simulink model "water_hopper_biped_FCPG_split"  (Simulink 8.0)
settings: Solver=ode23t  StartTime=0.0  StopTime=3  MaxStep=1e-3  RelTol=1e-3
values from neighbouring files (symbols this model uses):
  alpha = 30    [SimParam_FCPG.m]
  C_d = 0.703    [SimParam_FCPG.m]
  density = 1000    [SimParam_FCPG.m]
  freq = 60    [SimParam_FCPG.m]
  g = 9.81    [SimParam_FCPG.m]
  leg_length = 0.06    [SimParam_FCPG.m]
  mass = 0.05    [SimParam_FCPG.m]
  S1 = pi*r1^2    (= 0.00125663706144)    [SimParam_FCPG.m]
  S2 = pi*r2^2    (= 7.85398163397e-05)    [SimParam_FCPG.m]
  tau = 0.001    [SimParam_FCPG.m]
undefined symbols (not defined in the file): amp, RL_lag, y_0
libraries: mblibv1 x16, simulink x1
settings Model: Creator=Metti  LastModifiedBy=Metti
settings SolverCC: ZeroCrossControl=DisableAll
settings DataIOCC: SignalLoggingSaveFormat=ModelDataLogs
settings DebuggingCC: FcnCallInpInsideContextMsg=EnableAllAsWarning
settings ConfigurationSet: Description=SimMechanics 2G

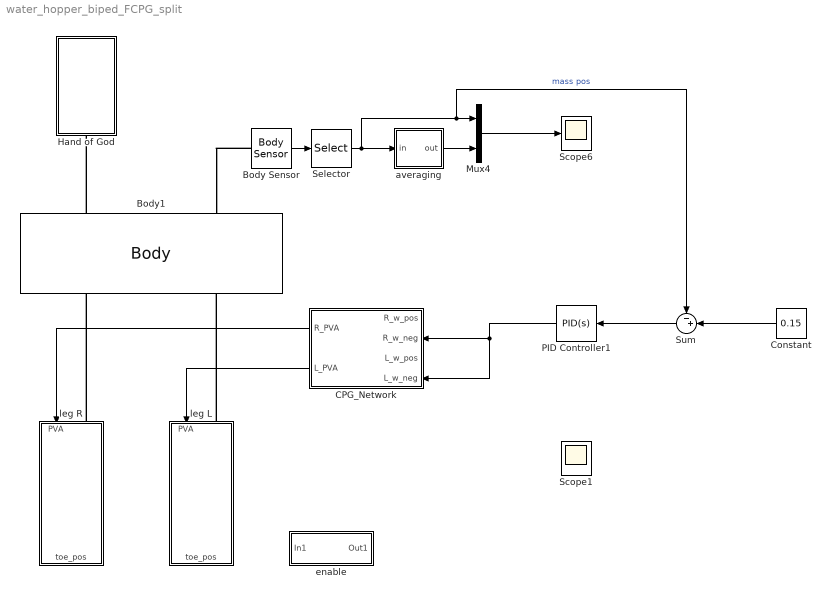
== system water_hopper_biped_FCPG_split ==
  Body Sensor : mblibv1/Sensors &  Actuators/Body Sensor  UpdateFromCAD=off  PhysicalDomain=Mechanical  PortType=blob  Muxed=on  Pose=off  Angle=on  AngleUnits=deg  ArcVelocity=off  ArcVelocityUnits=deg/s  ArcAcceleration=off  ArcAccelerationUnits=deg/s^2  CoordPosition=on  CoordPositionUnits=m  Velocity=off  VelocityUnits=m/s  Acceleration=off  AccelerationUnits=m/s^2  Quaternion=on  QuaternionDT=off  QuaternionDDT=off  QuaternionUnits=off  OutputVector=[1]  ActiveIO=on  Width=3  DialogClass=MechanicalSensorBlock  ReferenceFrame=Absolute (World)
  Body1 : mblibv1/Bodies/Body  LConnTagsString=CS1|CS2  RConnTagsString=CS3|CS4  UpdateFromCAD=off  DialogClass=MechanicalBodyBlock  Mass=mass  MassUnits=kg  InertiaUnits=kg*m^2  Inertia=eye(3)  Shape=Cylinder  ShapeDims=[1 1]  ShapeUnits=m  ShapeUse=false  Density=1  DensityUnits=kg/m^3  DensityUse=false  GraphicsMode=MACHINE_DEFAULT  BodyColorSelMode=MACHINE_DEFAULT  BodyColor=[1 0 0]  AttachedToCS=CG  CG=Left$CG$[0 0 0]$WORLD$WORLD$m$[0 0 0]$Euler X-Y-Z$deg$WORLD$false$none  WorkingFrames=Left$CS1$[0 0 0]$CG$CG$m$[0 0 0]$Euler X-Y-Z$deg$WORLD$true$none#Left$CS2$[0 0 0]$CG$CG$m$[0 0 0]$Euler X-Y-Z$deg$WORLD$true$none#Right$CS3$[0 0 0]$CG$CG$m$[0 0 0]$Euler X-Y-Z$deg$WORLD$true$none#Right$CS4$[0 0 0]$CG$CG$m$[0 0 0]$Euler X-Y-Z$deg$WORLD$true$none  CGPos=[0 0 0]  CGRot=[0 0 0]  CS0Pos=[]  CS0Rot=[]  CS1Pos=[0 0 0]  CS1Rot=[0 0 0]  CS2Pos=[0 0 0]  CS2Rot=[0 0 0]  CS3Pos=[0 0 0]  CS3Rot=[0 0 0]  CS4Pos=[0 0 0]  CS4Rot=[0 0 0]  CS5Pos=[]  CS5Rot=[]  CS6Pos=[]  CS6Rot=[]  CS7Pos=[]  CS7Rot=[]  CS8Pos=[]  CS8Rot=[]  CS9Pos=[]  CS9Rot=[]  CS10Pos=[]  CS10Rot=[]  CS11Pos=[]  CS11Rot=[]  CS12Pos=[]  CS12Rot=[]  CS13Pos=[]  CS13Rot=[]  CS14Pos=[]  CS14Rot=[]  CS15Pos=[]  CS15Rot=[]  CS16Pos=[]  CS16Rot=[]  CS17Pos=[]  CS17Rot=[]  CS18Pos=[]  CS18Rot=[]  CS19Pos=[]  CS19Rot=[]  CS20Pos=[]  CS20Rot=[]
  CPG_Network : Subsystem
  Constant : Constant  Value=0.15
  Hand of God : Subsystem
  Mux4 : Mux  Inputs=2
  PID Controller1 : simulink/Continuous/PID Controller  Controller=PID  TimeDomain=Continuous-time  SampleTime=1  IntegratorMethod=Forward Euler  FilterMethod=Forward Euler  Form=Parallel  P=100  I=0  D=0  N=100  InitialConditionSource=internal  InitialConditionForIntegrator=0  InitialConditionForFilter=0  ExternalReset=none  LimitOutput=off  UpperSaturationLimit=inf  LowerSaturationLimit=-inf  LinearizeAsGain=on  AntiWindupMode=none  Kb=1  TrackingMode=off  Kt=1  PParamMin=[]  PParamMax=[]  IParamMin=[]  IParamMax=[]  DParamMin=[]  DParamMax=[]  NParamMin=[]  NParamMax=[]  KbParamMin=[]  KbParamMax=[]  KtParamMin=[]  KtParamMax=[]  POutMin=[]  POutMax=[]  IOutMin=[]  IOutMax=[]  DOutMin=[]  DOutMax=[]  NOutMin=[]  NOutMax=[]  KbOutMin=[]  KbOutMax=[]  KtOutMin=[]  KtOutMax=[]  IntegratorOutMin=[]  IntegratorOutMax=[]  FilterOutMin=[]  FilterOutMax=[]  SumOutMin=[]  SumOutMax=[]  SumI1OutMin=[]  SumI1OutMax=[]  SumI2OutMin=[]  SumI2OutMax=[]  SumI3OutMin=[]  SumI3OutMax=[]  SumDOutMin=[]  SumDOutMax=[]  SaturationOutMin=[]  SaturationOutMax=[]  IntegratorContinuousStateAttributes=''  IntegratorStateMustResolveToSignalObject=off  IntegratorRTWStateStorageClass=Auto  FilterContinuousStateAttributes=''  FilterStateMustResolveToSignalObject=off  FilterRTWStateStorageClass=Auto
  Scope1 : Scope
      settings: YMin=0.066  YMax=0.079  SaveName=ball_position1
  Scope6 : Scope
      settings: YMin=0.066  YMax=0.079  SaveName=ball_position
  Selector : Selector  InputPortWidth=3  IndexOptions=Index vector (dialog)  Indices=[2]  OutputSizes=1
  Sum : Sum  Inputs=-+|
  averaging : Subsystem  mask{T_win=2*pi/freq/2, x_init=y_0}
      mask prompts: T_win "window (s)"; x_init "Initial condition"
  enable : Subsystem
  leg L : Subsystem
  leg R : Subsystem
  wires:
  Body Sensor/1 -> Selector/1
  Selector/1 -> averaging/1(in), Sum/1, Mux4/1  "mass pos"
  Mux4/1 -> Scope6/1
  CPG_Network/1(R_PVA) -> leg R/1(PVA)
  CPG_Network/2(L_PVA) -> leg L/1(PVA)
  Sum/1 -> PID Controller1/1
  averaging/1(out) -> Mux4/2
  Constant/1 -> Sum/2
  PID Controller1/1 -> CPG_Network/4(L_w_neg), CPG_Network/2(R_w_neg)
  connections:
  Body Sensor/LConn1 -- Body1/LConn2
  leg R/LConn1 -- Body1/RConn1
  Body1/LConn1 -- Hand of God/LConn1
  leg L/LConn1 -- Body1/RConn2

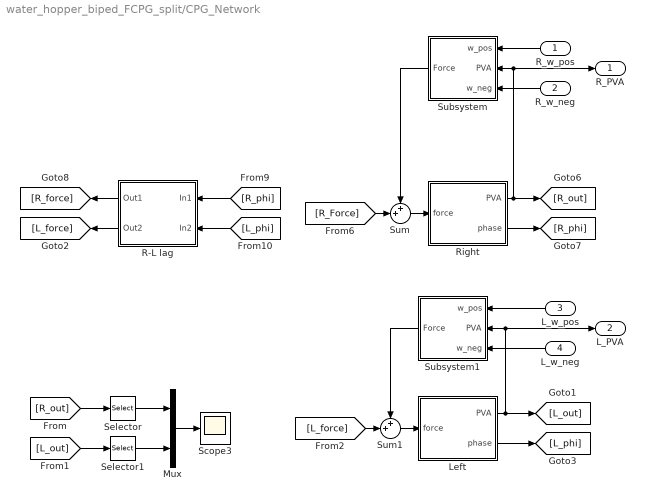
== system water_hopper_biped_FCPG_split/CPG_Network ==
  R_w_neg : Inport  Port=2
  L_w_pos : Inport  Port=3
  L_w_neg : Inport  Port=4
  Left : Subsystem  mask{Amp=amp, Offset=0, init_phi=pi}
      mask prompts: Amp "Amplitude"; init_phi "Initial Phase"
  Mux : Mux  Inputs=2
  R-L lag : Subsystem  mask{d_phase=RL_lag, coupling_weight=2}
      mask prompts: d_phase "Phase Lag"; coupling_weight "Coupling Weight"
  Right : Subsystem  mask{Amp=amp, Offset=0, init_phi=0}
      mask prompts: Amp "Amplitude"; init_phi "Initial Phase"
  Scope3 : Scope
      settings: TimeRange=10  YMin=0  YMax=2  SaveName=Output
  Selector : Selector  InputPortWidth=3  IndexOptions=Index vector (dialog)  Indices=[1]  OutputSizes=1
  Selector1 : Selector  InputPortWidth=3  IndexOptions=Index vector (dialog)  Indices=[1]  OutputSizes=1
  Sum : Sum  Inputs=++|
  Sum1 : Sum  Inputs=++|
  R_w_pos : Inport
  Subsystem : Subsystem
  Subsystem1 : Subsystem
  R_PVA : Outport
  L_PVA : Outport  Port=2
  wires:
  Mux/1 -> Scope3/1
  Left/2(phase) -> [L_phi]
  Right/2(phase) -> [R_phi]
  [L_phi] -> R-L lag/2(In2)
  [R_phi] -> R-L lag/1(In1)
  R-L lag/1(Out1) -> [R_force]
  R-L lag/2(Out2) -> [L_force]
  Right/1(PVA) -> R_PVA/1, Subsystem/2(PVA), [R_out]
  [L_force] -> Sum1/2
  Sum1/1 -> Left/1(force)
  Sum/1 -> Right/1(force)
  [R_Force] -> Sum/2
  [L_out] -> Selector1/1
  Selector1/1 -> Mux/2
  Selector/1 -> Mux/1
  [R_out] -> Selector/1
  R_w_pos/1 -> Subsystem/1(w_pos)
  R_w_neg/1 -> Subsystem/3(w_neg)
  Subsystem/1(Force) -> Sum/1
  L_w_pos/1 -> Subsystem1/1(w_pos)
  L_w_neg/1 -> Subsystem1/3(w_neg)
  Left/1(PVA) -> Subsystem1/2(PVA), L_PVA/1, [L_out]
  Subsystem1/1(Force) -> Sum1/1

== system water_hopper_biped_FCPG_split/Hand of God ==
  Ground : mblibv1/Bodies/Ground  UpdateFromCAD=off  LeftPortType=env  RightPortType=workingframe  PhysicalDomain=Mechanical  DialogClass=GroundBlock  CoordPosition=[0 0 0]  CoordPositionUnits=m  StateVectorMgrId=2  MachineId=[3 0]  ShowEnvPort=on
  Joint Initial Condition : mblibv1/Sensors &  Actuators/Joint Initial Condition  UpdateFromCAD=off  LeftPortType=blob  RightPortType=blob  PhysicalDomain=mechanical  DialogClass=InitialConditionBlock  InitialConditions=P1$true$y_0$m$deg$0$m/s$deg/s#P2$false$0$m$deg$0$m/s$deg/s#P3$false$0$m$deg$0$m/s$deg/s#R1$false$0$m$deg$0$m/s$deg/s#R2$false$0$m$deg$0$m/s$deg/s#R3$false$0$m$deg$0$m/s$deg/s#S$false$0$m$deg$0$m/s$deg/s  P1PIC=y_0  P1VIC=0  P2PIC=0  P2VIC=0  P3PIC=0  P3VIC=0  R1PIC=0  R1VIC=0  R2PIC=0  R2VIC=0  R3PIC=0  R3VIC=0  SPIC=0  SVIC=0
  Machine Environment : mblibv1/Bodies/Machine Environment  PortType=env  PhysicalDomain=Mechanical  DialogTemplateClass=MECH.MachineEnvironment  SyncWhenCopied=off  Gravity=[0 -g 0]  GravityUnits=m/s^2  GravityAsSignal=off  Dimensionality=Auto-detect  AnalysisType=Forward dynamics  LinearAssemblyTolerance=1e-3  LinearAssemblyToleranceUnits=m  AngularAssemblyTolerance=1e-3  AngularAssemblyToleranceUnits=rad  ConstraintSolverType=Stabilizing  ConstraintRelTolerance=1e-4  ConstraintAbsTolerance=1e-4  UseRobustSingularityHandling=off  RedundancyAnalysisToleranceType=Automatically select tolerance  RedundancyAnalysisTolerance=1e-14  StatePerturbationType=Fixed  PerturbationSize=1e-5  VisualizeMachine=on  BodyVisualizationType=Use model default body geometries  BodyColorSelMode=Use model default  DefaultBodyColor=[1 0 0]
  Prismatic : mblibv1/Joints/Prismatic  LConnTagsString=__newl0|SA1  RConnTagsString=__newr0  UpdateFromCAD=off  NumSAPorts=1  CutJoint=off  MarkAsCut=off  Primitives=prismatic  PrimitiveProps=P1$World$[0 1 0]$prismatic  DialogClass=JointBlock  P1Axis=[0 1 0]
  Conn1 : PMIOPort  Port=1  Side=Left
  connections:
  Conn1/RConn1 -- Prismatic/RConn1
  Machine Environment/RConn1 -- Ground/LConn1
  Ground/RConn1 -- Prismatic/LConn1
  Joint Initial Condition/RConn1 -- Prismatic/LConn2

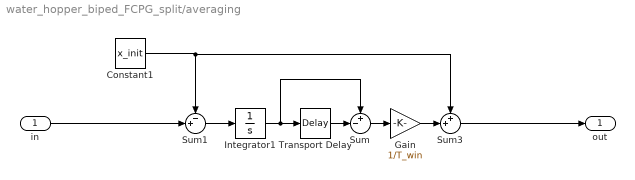
== system water_hopper_biped_FCPG_split/averaging ==
  in : Inport
  Constant1 : Constant  Value=x_init
  Gain : Gain  Gain=1/T_win
  Integrator1 : Integrator
  Sum : Sum  Inputs=+-|
  Sum1 : Sum  Inputs=-+|
  Sum3 : Sum  Inputs=++|
  Transport Delay : TransportDelay  DelayTime=T_win
  out : Outport
  wires:
  in/1 -> Sum1/2
  Gain/1 -> Sum3/2
  Constant1/1 -> Sum3/1, Sum1/1
  Sum1/1 -> Integrator1/1
  Transport Delay/1 -> Sum/2
  Integrator1/1 -> Sum/1, Transport Delay/1
  Sum3/1 -> out/1
  Sum/1 -> Gain/1

== system water_hopper_biped_FCPG_split/enable ==
  In1 : Inport
  Constant1 : Constant
  Derivative : Derivative
  Gain : Gain  Gain=.5
  Sign : Signum
  Sum1 : Sum  Inputs=|-+
  Out1 : Outport
  wires:
  Derivative/1 -> Sign/1
  Constant1/1 -> Sum1/2
  Sign/1 -> Sum1/1
  Gain/1 -> Out1/1
  In1/1 -> Derivative/1
  Sum1/1 -> Gain/1

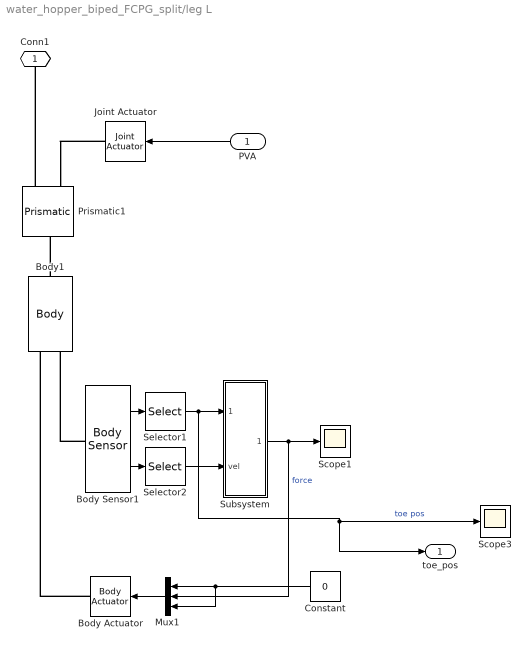
== system water_hopper_biped_FCPG_split/leg L ==
  PVA : Inport
  Body Actuator : mblibv1/Sensors &  Actuators/Body Actuator  UpdateFromCAD=off  PhysicalDomain=Mechanical  PortType=blob  ActuationStyle=Force  AngleUnits=deg  ArcVelocityUnits=deg/s  ArcAccelerationUnits=deg/s^2  CoordPositionUnits=m  VelocityUnits=m/s  AccelerationUnits=m/s^2  ForceUnits=N  TorqueUnits=N-m  ActiveIO=on  Width=3  DialogClass=MechanicalActuatorBlock  ReferenceFrame=Absolute (World)  Angle=off  CoordPosition=on  Force=on  Torque=off
  Body Sensor1 : mblibv1/Sensors &  Actuators/Body Sensor  UpdateFromCAD=off  PhysicalDomain=Mechanical  PortType=blob  Muxed=off  Pose=off  Angle=on  AngleUnits=deg  ArcVelocity=off  ArcVelocityUnits=deg/s  ArcAcceleration=off  ArcAccelerationUnits=deg/s^2  CoordPosition=on  CoordPositionUnits=m  Velocity=on  VelocityUnits=m/s  Acceleration=off  AccelerationUnits=m/s^2  Quaternion=on  QuaternionDT=off  QuaternionDDT=off  QuaternionUnits=off  OutputVector=[1]  ActiveIO=on  Width=6  DialogClass=MechanicalSensorBlock  ReferenceFrame=Absolute (World)
  Body1 : mblibv1/Bodies/Body  LConnTagsString=CS1  RConnTagsString=CS2|CS3  UpdateFromCAD=off  DialogClass=MechanicalBodyBlock  Mass=0  MassUnits=kg  InertiaUnits=kg*m^2  Inertia=zeros(3)  Shape=Cylinder  ShapeDims=[1 1]  ShapeUnits=m  ShapeUse=false  Density=1  DensityUnits=kg/m^3  DensityUse=false  GraphicsMode=MACHINE_DEFAULT  BodyColorSelMode=MACHINE_DEFAULT  BodyColor=[1 0 0]  AttachedToCS=CG  CG=Left$CG$[0 -leg_length 0]$CS1$CS1$m$[0 0 0]$Euler X-Y-Z$deg$WORLD$false$none  WorkingFrames=Left$CS1$[0 0 0]$Adjoining$Adjoining$m$[0 0 0]$Euler X-Y-Z$deg$WORLD$true$none#Right$CS2$[0 -leg_length 0]$CS1$CS1$m$[0 0 0]$Euler X-Y-Z$deg$WORLD$true$none#Right$CS3$[0 -leg_length 0]$CS1$CS1$m$[0 0 0]$Euler X-Y-Z$deg$WORLD$true$none  CGPos=[0 -leg_length 0]  CGRot=[0 0 0]  CS0Pos=[]  CS0Rot=[]  CS1Pos=[0 0 0]  CS1Rot=[0 0 0]  CS2Pos=[0 -leg_length 0]  CS2Rot=[0 0 0]  CS3Pos=[0 -leg_length 0]  CS3Rot=[0 0 0]  CS4Pos=[]  CS4Rot=[]  CS5Pos=[]  CS5Rot=[]  CS6Pos=[]  CS6Rot=[]  CS7Pos=[]  CS7Rot=[]  CS8Pos=[]  CS8Rot=[]  CS9Pos=[]  CS9Rot=[]  CS10Pos=[]  CS10Rot=[]  CS11Pos=[]  CS11Rot=[]  CS12Pos=[]  CS12Rot=[]  CS13Pos=[]  CS13Rot=[]  CS14Pos=[]  CS14Rot=[]  CS15Pos=[]  CS15Rot=[]  CS16Pos=[]  CS16Rot=[]  CS17Pos=[]  CS17Rot=[]  CS18Pos=[]  CS18Rot=[]  CS19Pos=[]  CS19Rot=[]  CS20Pos=[]  CS20Rot=[]
  Constant : Constant  Value=0
  Joint Actuator : mblibv1/Sensors &  Actuators/Joint Actuator  UpdateFromCAD=off  PhysicalDomain=Mechanical  PortType=blob  ActuationStyle=Motion  AngleUnits=deg  ArcVelocityUnits=deg/s  ArcAccelerationUnits=deg/s^2  CoordPositionUnits=m  VelocityUnits=m/s  AccelerationUnits=m/s^2  ForceUnits=N  TorqueUnits=N*m  ActiveIO=on  Width=3  DialogClass=MechanicalActuatorBlock  Primitive=P1  ReferenceFrame=Absolute (World)
  Mux1 : Mux  Inputs=3
  Prismatic1 : mblibv1/Joints/Prismatic  LConnTagsString=__newl0|SA1  RConnTagsString=__newr0  UpdateFromCAD=off  NumSAPorts=1  CutJoint=off  MarkAsCut=off  Primitives=prismatic  PrimitiveProps=P1$World$[0 1 0]$prismatic  DialogClass=JointBlock  P1Axis=[0 1 0]
  Scope1 : Scope
      settings: SaveName=force_L
  Scope3 : Scope
      settings: SaveName=toe_position_L
  Selector1 : Selector  InputPortWidth=3  IndexOptions=Index vector (dialog)  Indices=[2]  OutputSizes=1
  Selector2 : Selector  InputPortWidth=3  IndexOptions=Index vector (dialog)  Indices=[2]  OutputSizes=1
  Subsystem : Subsystem
  Conn1 : PMIOPort  Port=1  Side=Left
  toe_pos : Outport
  wires:
  PVA/1 -> Joint Actuator/1
  Constant/1 -> Mux1/3, Mux1/1
  Mux1/1 -> Body Actuator/1
  Subsystem/1(force) -> Mux1/2, Scope1/1  "force"
  Selector2/1 -> Subsystem/2(vel)
  Selector1/1 -> toe_pos/1, Scope3/1, Subsystem/1(pos)  "toe pos"
  Body Sensor1/2 -> Selector2/1
  Body Sensor1/1 -> Selector1/1
  connections:
  Joint Actuator/RConn1 -- Prismatic1/LConn2
  Prismatic1/LConn1 -- Conn1/RConn1
  Body Sensor1/LConn1 -- Body1/RConn2
  Body Actuator/RConn1 -- Body1/RConn1
  Body1/LConn1 -- Prismatic1/RConn1

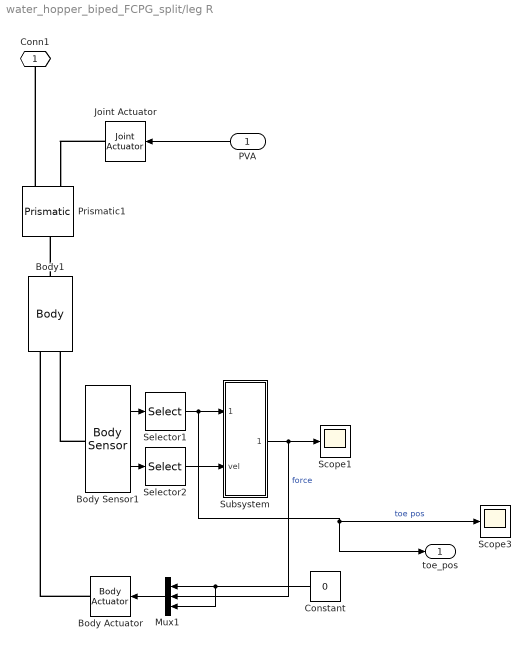
== system water_hopper_biped_FCPG_split/leg R ==
  PVA : Inport
  Body Actuator : mblibv1/Sensors &  Actuators/Body Actuator  UpdateFromCAD=off  PhysicalDomain=Mechanical  PortType=blob  ActuationStyle=Force  AngleUnits=deg  ArcVelocityUnits=deg/s  ArcAccelerationUnits=deg/s^2  CoordPositionUnits=m  VelocityUnits=m/s  AccelerationUnits=m/s^2  ForceUnits=N  TorqueUnits=N-m  ActiveIO=on  Width=3  DialogClass=MechanicalActuatorBlock  ReferenceFrame=Absolute (World)  Angle=off  CoordPosition=on  Force=on  Torque=off
  Body Sensor1 : mblibv1/Sensors &  Actuators/Body Sensor  UpdateFromCAD=off  PhysicalDomain=Mechanical  PortType=blob  Muxed=off  Pose=off  Angle=on  AngleUnits=deg  ArcVelocity=off  ArcVelocityUnits=deg/s  ArcAcceleration=off  ArcAccelerationUnits=deg/s^2  CoordPosition=on  CoordPositionUnits=m  Velocity=on  VelocityUnits=m/s  Acceleration=off  AccelerationUnits=m/s^2  Quaternion=on  QuaternionDT=off  QuaternionDDT=off  QuaternionUnits=off  OutputVector=[1]  ActiveIO=on  Width=6  DialogClass=MechanicalSensorBlock  ReferenceFrame=Absolute (World)
  Body1 : mblibv1/Bodies/Body  LConnTagsString=CS1  RConnTagsString=CS2|CS3  UpdateFromCAD=off  DialogClass=MechanicalBodyBlock  Mass=0  MassUnits=kg  InertiaUnits=kg*m^2  Inertia=zeros(3)  Shape=Cylinder  ShapeDims=[1 1]  ShapeUnits=m  ShapeUse=false  Density=1  DensityUnits=kg/m^3  DensityUse=false  GraphicsMode=MACHINE_DEFAULT  BodyColorSelMode=MACHINE_DEFAULT  BodyColor=[1 0 0]  AttachedToCS=CG  CG=Left$CG$[0 -leg_length 0]$CS1$CS1$m$[0 0 0]$Euler X-Y-Z$deg$WORLD$false$none  WorkingFrames=Left$CS1$[0 0 0]$Adjoining$Adjoining$m$[0 0 0]$Euler X-Y-Z$deg$WORLD$true$none#Right$CS2$[0 -leg_length 0]$CS1$CS1$m$[0 0 0]$Euler X-Y-Z$deg$WORLD$true$none#Right$CS3$[0 -leg_length 0]$CS1$CS1$m$[0 0 0]$Euler X-Y-Z$deg$WORLD$true$none  CGPos=[0 -leg_length 0]  CGRot=[0 0 0]  CS0Pos=[]  CS0Rot=[]  CS1Pos=[0 0 0]  CS1Rot=[0 0 0]  CS2Pos=[0 -leg_length 0]  CS2Rot=[0 0 0]  CS3Pos=[0 -leg_length 0]  CS3Rot=[0 0 0]  CS4Pos=[]  CS4Rot=[]  CS5Pos=[]  CS5Rot=[]  CS6Pos=[]  CS6Rot=[]  CS7Pos=[]  CS7Rot=[]  CS8Pos=[]  CS8Rot=[]  CS9Pos=[]  CS9Rot=[]  CS10Pos=[]  CS10Rot=[]  CS11Pos=[]  CS11Rot=[]  CS12Pos=[]  CS12Rot=[]  CS13Pos=[]  CS13Rot=[]  CS14Pos=[]  CS14Rot=[]  CS15Pos=[]  CS15Rot=[]  CS16Pos=[]  CS16Rot=[]  CS17Pos=[]  CS17Rot=[]  CS18Pos=[]  CS18Rot=[]  CS19Pos=[]  CS19Rot=[]  CS20Pos=[]  CS20Rot=[]
  Constant : Constant  Value=0
  Joint Actuator : mblibv1/Sensors &  Actuators/Joint Actuator  UpdateFromCAD=off  PhysicalDomain=Mechanical  PortType=blob  ActuationStyle=Motion  AngleUnits=deg  ArcVelocityUnits=deg/s  ArcAccelerationUnits=deg/s^2  CoordPositionUnits=m  VelocityUnits=m/s  AccelerationUnits=m/s^2  ForceUnits=N  TorqueUnits=N*m  ActiveIO=on  Width=3  DialogClass=MechanicalActuatorBlock  Primitive=P1  ReferenceFrame=Absolute (World)
  Mux1 : Mux  Inputs=3
  Prismatic1 : mblibv1/Joints/Prismatic  LConnTagsString=__newl0|SA1  RConnTagsString=__newr0  UpdateFromCAD=off  NumSAPorts=1  CutJoint=off  MarkAsCut=off  Primitives=prismatic  PrimitiveProps=P1$World$[0 1 0]$prismatic  DialogClass=JointBlock  P1Axis=[0 1 0]
  Scope1 : Scope
      settings: SaveName=force_L
  Scope3 : Scope
      settings: SaveName=toe_position_L
  Selector1 : Selector  InputPortWidth=3  IndexOptions=Index vector (dialog)  Indices=[2]  OutputSizes=1
  Selector2 : Selector  InputPortWidth=3  IndexOptions=Index vector (dialog)  Indices=[2]  OutputSizes=1
  Subsystem : Subsystem
  Conn1 : PMIOPort  Port=1  Side=Left
  toe_pos : Outport
  wires:
  Body Sensor1/1 -> Selector1/1
  Body Sensor1/2 -> Selector2/1
  Selector1/1 -> Subsystem/1(pos), Scope3/1, toe_pos/1  "toe pos"
  Selector2/1 -> Subsystem/2(vel)
  Subsystem/1(force) -> Scope1/1, Mux1/2  "force"
  Mux1/1 -> Body Actuator/1
  Constant/1 -> Mux1/1, Mux1/3
  PVA/1 -> Joint Actuator/1
  connections:
  Body1/LConn1 -- Prismatic1/RConn1
  Body Actuator/RConn1 -- Body1/RConn1
  Body Sensor1/LConn1 -- Body1/RConn2
  Prismatic1/LConn1 -- Conn1/RConn1
  Joint Actuator/RConn1 -- Prismatic1/LConn2

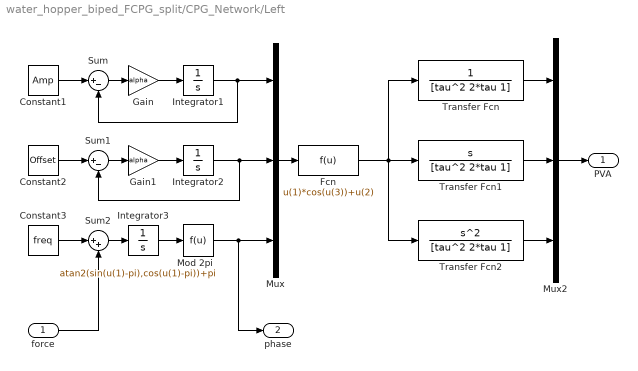
== system water_hopper_biped_FCPG_split/CPG_Network/Left ==
  force : Inport
  Constant1 : Constant  Value=Amp
  Constant2 : Constant  Value=Offset
  Constant3 : Constant  Value=freq
  Fcn : Fcn  Expr=u(1)*cos(u(3))+u(2)
  Gain : Gain  Gain=alpha
  Gain1 : Gain  Gain=alpha
  Integrator1 : Integrator
  Integrator2 : Integrator
  Integrator3 : Integrator  InitialCondition=init_phi + 0.01*rand
  Mod 2pi : Fcn  Expr=atan2(sin(u(1)-pi),cos(u(1)-pi))+pi
  Mux : Mux  Inputs=3
  Mux2 : Mux  Inputs=3
  Sum : Sum  Inputs=|+-
  Sum1 : Sum  Inputs=|+-
  Sum2 : Sum  Inputs=|++
  Transfer Fcn : TransferFcn  Denominator=[tau^2 2*tau 1]
  Transfer Fcn1 : TransferFcn  Numerator=[1 0]  Denominator=[tau^2 2*tau 1]
  Transfer Fcn2 : TransferFcn  Numerator=[1 0 0]  Denominator=[tau^2 2*tau 1]
  PVA : Outport
  phase : Outport  Port=2
  wires:
  Mux2/1 -> PVA/1
  Fcn/1 -> Transfer Fcn1/1, Transfer Fcn/1, Transfer Fcn2/1
  Transfer Fcn1/1 -> Mux2/2
  Transfer Fcn/1 -> Mux2/1
  Transfer Fcn2/1 -> Mux2/3
  force/1 -> Sum2/2
  Sum2/1 -> Integrator3/1
  Constant3/1 -> Sum2/1
  Integrator3/1 -> Mod 2pi/1
  Mod 2pi/1 -> Mux/3, phase/1
  Mux/1 -> Fcn/1
  Gain1/1 -> Integrator2/1
  Constant2/1 -> Sum1/1
  Integrator2/1 -> Mux/2, Sum1/2
  Sum1/1 -> Gain1/1
  Gain/1 -> Integrator1/1
  Constant1/1 -> Sum/1
  Integrator1/1 -> Mux/1, Sum/2
  Sum/1 -> Gain/1

== system water_hopper_biped_FCPG_split/CPG_Network/R-L lag ==
  In1 : Inport
  In2 : Inport  Port=2
  Constant : Constant  Value=d_phase
  Gain : Gain  Gain=-1
  Sum : Sum  Inputs=--+
  sin : Fcn  Expr=coupling_weight*sin(u(1))
  Out1 : Outport
  Out2 : Outport  Port=2
  wires:
  Sum/1 -> sin/1
  sin/1 -> Gain/1, Out1/1
  Constant/1 -> Sum/2
  In1/1 -> Sum/1
  In2/1 -> Sum/3
  Gain/1 -> Out2/1

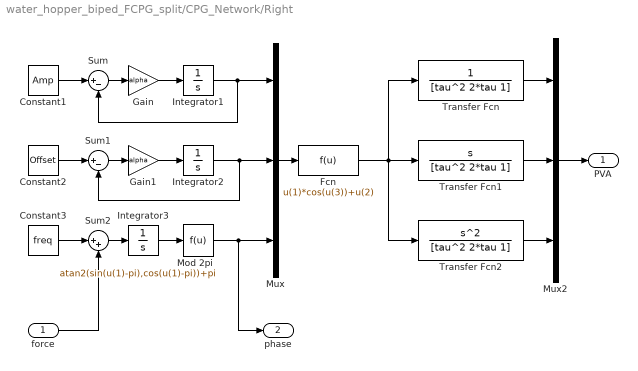
== system water_hopper_biped_FCPG_split/CPG_Network/Right ==
  force : Inport
  Constant1 : Constant  Value=Amp
  Constant2 : Constant  Value=Offset
  Constant3 : Constant  Value=freq
  Fcn : Fcn  Expr=u(1)*cos(u(3))+u(2)
  Gain : Gain  Gain=alpha
  Gain1 : Gain  Gain=alpha
  Integrator1 : Integrator
  Integrator2 : Integrator
  Integrator3 : Integrator  InitialCondition=init_phi + 0.01*rand
  Mod 2pi : Fcn  Expr=atan2(sin(u(1)-pi),cos(u(1)-pi))+pi
  Mux : Mux  Inputs=3
  Mux2 : Mux  Inputs=3
  Sum : Sum  Inputs=|+-
  Sum1 : Sum  Inputs=|+-
  Sum2 : Sum  Inputs=|++
  Transfer Fcn : TransferFcn  Denominator=[tau^2 2*tau 1]
  Transfer Fcn1 : TransferFcn  Numerator=[1 0]  Denominator=[tau^2 2*tau 1]
  Transfer Fcn2 : TransferFcn  Numerator=[1 0 0]  Denominator=[tau^2 2*tau 1]
  PVA : Outport
  phase : Outport  Port=2
  wires:
  Sum/1 -> Gain/1
  Integrator1/1 -> Sum/2, Mux/1
  Constant1/1 -> Sum/1
  Gain/1 -> Integrator1/1
  Sum1/1 -> Gain1/1
  Integrator2/1 -> Sum1/2, Mux/2
  Constant2/1 -> Sum1/1
  Gain1/1 -> Integrator2/1
  Mux/1 -> Fcn/1
  Mod 2pi/1 -> phase/1, Mux/3
  Integrator3/1 -> Mod 2pi/1
  Constant3/1 -> Sum2/1
  Sum2/1 -> Integrator3/1
  force/1 -> Sum2/2
  Transfer Fcn2/1 -> Mux2/3
  Transfer Fcn/1 -> Mux2/1
  Transfer Fcn1/1 -> Mux2/2
  Fcn/1 -> Transfer Fcn2/1, Transfer Fcn/1, Transfer Fcn1/1
  Mux2/1 -> PVA/1

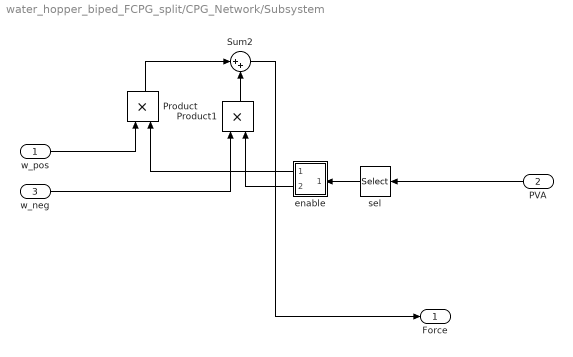
== system water_hopper_biped_FCPG_split/CPG_Network/Subsystem ==
  w_pos : Inport
  PVA : Inport  Port=2
  w_neg : Inport  Port=3
  Product : Product  RndMeth=Zero
  Product1 : Product  RndMeth=Zero
  Sum2 : Sum  Inputs=|++
  enable : Subsystem
  sel : Selector  InputPortWidth=3  IndexOptions=Index vector (dialog)  Indices=[2]  OutputSizes=1
  Force : Outport
  wires:
  Product/1 -> Sum2/1
  w_pos/1 -> Product/1
  w_neg/1 -> Product1/1
  Product1/1 -> Sum2/2
  PVA/1 -> sel/1
  enable/1(pos) -> Product/2
  enable/2(neg) -> Product1/2
  Sum2/1 -> Force/1
  sel/1 -> enable/1(in)

== system water_hopper_biped_FCPG_split/CPG_Network/Subsystem1 ==
  w_pos : Inport
  PVA : Inport  Port=2
  w_neg : Inport  Port=3
  Product : Product  RndMeth=Zero
  Product1 : Product  RndMeth=Zero
  Sum2 : Sum  Inputs=|++
  enable : Subsystem
  sel : Selector  InputPortWidth=3  IndexOptions=Index vector (dialog)  Indices=[2]  OutputSizes=1
  Force : Outport
  wires:
  Product/1 -> Sum2/1
  w_pos/1 -> Product/1
  w_neg/1 -> Product1/1
  Product1/1 -> Sum2/2
  PVA/1 -> sel/1
  enable/1(pos) -> Product/2
  enable/2(neg) -> Product1/2
  Sum2/1 -> Force/1
  sel/1 -> enable/1(in)

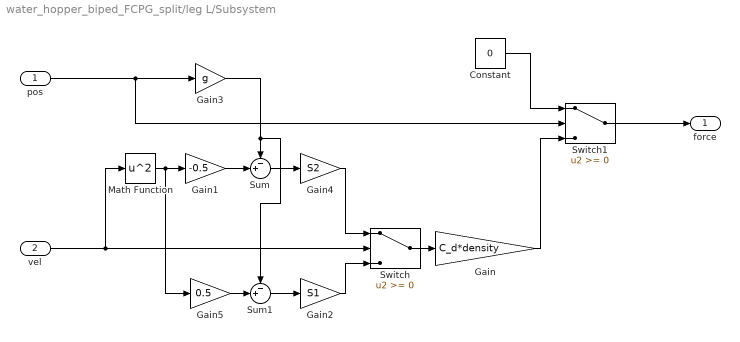
== system water_hopper_biped_FCPG_split/leg L/Subsystem ==
  pos : Inport
  vel : Inport  Port=2
  Constant : Constant  Value=0
  Gain : Gain  Gain=C_d*density
  Gain1 : Gain  Gain=-0.5
  Gain2 : Gain  Gain=S1
  Gain3 : Gain  Gain=g
  Gain4 : Gain  Gain=S2
  Gain5 : Gain  Gain=0.5
  Math Function : Math  Operator=square  SaturateOnIntegerOverflow=on
  Sum : Sum  Inputs=-+|
  Sum1 : Sum  Inputs=-+|
  Switch : Switch  ZeroCross=off
  Switch1 : Switch
  force : Outport
  wires:
  Gain5/1 -> Sum1/2
  Sum1/1 -> Gain2/1
  Constant/1 -> Switch1/1
  Gain/1 -> Switch1/3
  Switch1/1 -> force/1
  Switch/1 -> Gain/1
  Gain2/1 -> Switch/3
  Gain4/1 -> Switch/1
  Sum/1 -> Gain4/1
  Gain3/1 -> Sum1/1, Sum/1
  pos/1 -> Switch1/2, Gain3/1
  Gain1/1 -> Sum/2
  Math Function/1 -> Gain5/1, Gain1/1
  vel/1 -> Math Function/1, Switch/2

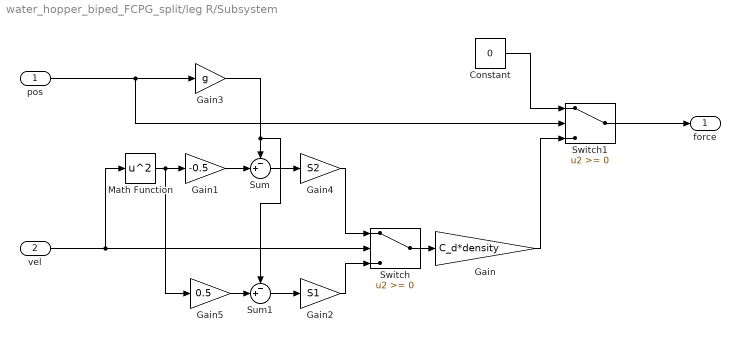
== system water_hopper_biped_FCPG_split/leg R/Subsystem ==
  pos : Inport
  vel : Inport  Port=2
  Constant : Constant  Value=0
  Gain : Gain  Gain=C_d*density
  Gain1 : Gain  Gain=-0.5
  Gain2 : Gain  Gain=S1
  Gain3 : Gain  Gain=g
  Gain4 : Gain  Gain=S2
  Gain5 : Gain  Gain=0.5
  Math Function : Math  Operator=square  SaturateOnIntegerOverflow=on
  Sum : Sum  Inputs=-+|
  Sum1 : Sum  Inputs=-+|
  Switch : Switch  ZeroCross=off
  Switch1 : Switch
  force : Outport
  wires:
  vel/1 -> Switch/2, Math Function/1
  Math Function/1 -> Gain1/1, Gain5/1
  Gain1/1 -> Sum/2
  pos/1 -> Gain3/1, Switch1/2
  Gain3/1 -> Sum/1, Sum1/1
  Sum/1 -> Gain4/1
  Gain4/1 -> Switch/1
  Gain2/1 -> Switch/3
  Switch/1 -> Gain/1
  Switch1/1 -> force/1
  Gain/1 -> Switch1/3
  Constant/1 -> Switch1/1
  Sum1/1 -> Gain2/1
  Gain5/1 -> Sum1/2

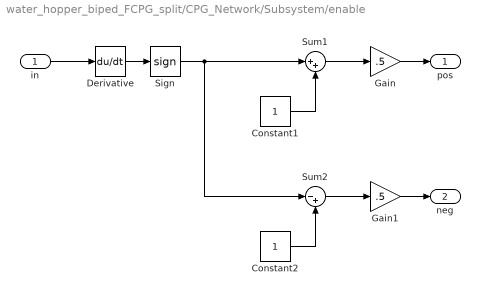
== system water_hopper_biped_FCPG_split/CPG_Network/Subsystem/enable ==
  in : Inport
  Constant1 : Constant
  Constant2 : Constant
  Derivative : Derivative
  Gain : Gain  Gain=.5
  Gain1 : Gain  Gain=.5
  Sign : Signum
  Sum1 : Sum  Inputs=|++
  Sum2 : Sum  Inputs=|-+
  pos : Outport
  neg : Outport  Port=2
  wires:
  Derivative/1 -> Sign/1
  Constant1/1 -> Sum1/2
  Sign/1 -> Sum2/1, Sum1/1
  Gain/1 -> pos/1
  in/1 -> Derivative/1
  Sum1/1 -> Gain/1
  Constant2/1 -> Sum2/2
  Gain1/1 -> neg/1
  Sum2/1 -> Gain1/1

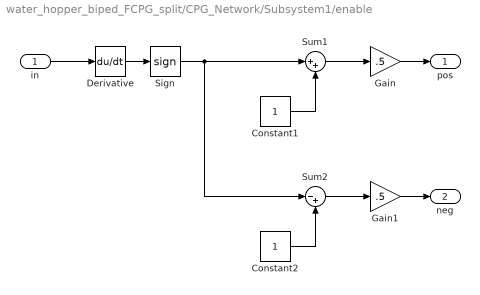
== system water_hopper_biped_FCPG_split/CPG_Network/Subsystem1/enable ==
  in : Inport
  Constant1 : Constant
  Constant2 : Constant
  Derivative : Derivative
  Gain : Gain  Gain=.5
  Gain1 : Gain  Gain=.5
  Sign : Signum
  Sum1 : Sum  Inputs=|++
  Sum2 : Sum  Inputs=|-+
  pos : Outport
  neg : Outport  Port=2
  wires:
  Derivative/1 -> Sign/1
  Constant1/1 -> Sum1/2
  Sign/1 -> Sum2/1, Sum1/1
  Gain/1 -> pos/1
  in/1 -> Derivative/1
  Sum1/1 -> Gain/1
  Constant2/1 -> Sum2/2
  Gain1/1 -> neg/1
  Sum2/1 -> Gain1/1
